simulink model "ProgrammingCalculator"  (R2021a)
settings: Solver=FixedStepDiscrete  StartTime=0.0  StopTime=10.0  RelTol=1e-3  EnableMultiTasking=on
libraries: simulink x6
settings Model: Creator=top one  LastModifiedBy=top one
settings DataIOCC: ReturnWorkspaceOutputs=off
settings OptimizationCC: DefaultParameterBehavior=Inlined  InlineInvariantSignals=on  EnableMemcpy=off  LifeSpan=1  EfficientTunableParamExpr=on
settings DebuggingCC: UnderspecifiedInitializationDetection=Classic  MergeDetectMultiDrivingBlocksExec=none  SFMachineParentedDataDiag=warning  ArithmeticOperatorsInVariantConditions=warning
settings ModelReferenceCC: PropagateSignalLabelsOutOfModel=off
settings SFSimCC: MATLABDynamicMemAlloc=off  CustomCodeUndefinedFunction=UseInterfaceOnly
settings RTWCC: SystemTargetFile=ert.tlc  GenCodeOnly=on  TemplateMakefile=ert_default_tmf  GenerateReport=on  IncludeHyperlinkInReport=on  LaunchReport=on  GenerateTraceInfo=on  GenerateTraceReport=on  GenerateTraceReportSl=on  GenerateTraceReportSf=on  GenerateTraceReportEml=on
settings CodeAppCC: ForceParamTrailComments=on  IgnoreCustomStorageClasses=off  OperatorAnnotations=on  SimulinkDataObjDesc=on  SFDataObjDesc=on  MATLABFcnDesc=on  InsertBlockDesc=on  StateflowObjectComments=on  MATLABSourceComments=on
settings ERTTargetCC: MultiwordLength=2048  GenerateSampleERTMain=on  InlinedParameterPlacement=NonHierarchical  ERTCustomFileTemplate=example_file_process.tlc

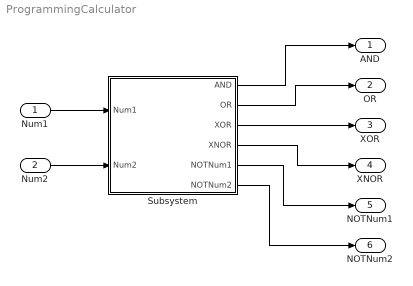
== system ProgrammingCalculator ==
  Num1 : Inport
  Num2 : Inport  Port=2
  Subsystem : Subsystem
  AND : Outport
  OR : Outport  Port=2
  XOR : Outport  Port=3
  XNOR : Outport  Port=4
  NOTNum1 : Outport  Port=5
  NOTNum2 : Outport  Port=6
  wires:
  Subsystem/1(AND) -> AND/1
  Subsystem/2(OR) -> OR/1
  Subsystem/3(XOR) -> XOR/1
  Subsystem/4(XNOR) -> XNOR/1
  Subsystem/5(NOTNum1) -> NOTNum1/1
  Subsystem/6(NOTNum2) -> NOTNum2/1
  Num2/1 -> Subsystem/2(Num2)
  Num1/1 -> Subsystem/1(Num1)

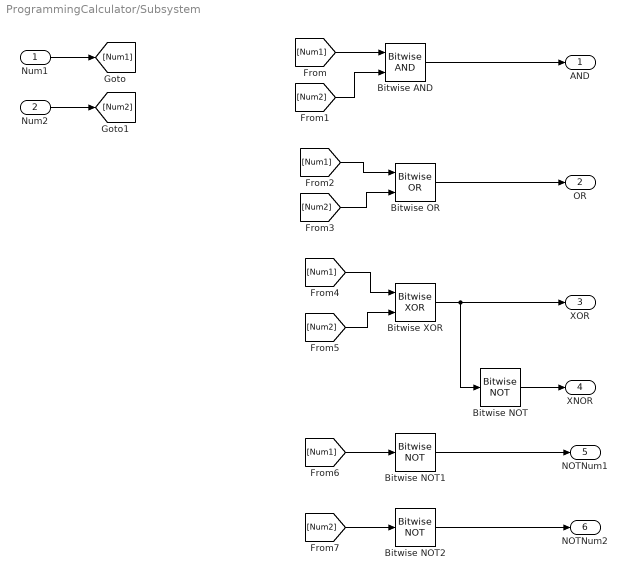
== system ProgrammingCalculator/Subsystem ==
  Num1 : Inport  OutDataTypeStr=uint8
  Num2 : Inport  Port=2  OutDataTypeStr=uint8
  Bitwise AND : simulink/Logic and Bit Operations/Bitwise Operator  logicop=AND  UseBitMask=off  NumInputPorts=2  BitMask=bin2dec('11011001')  BitMaskRealWorld=Stored Integer
  Bitwise NOT : simulink/Logic and Bit Operations/Bitwise Operator  logicop=NOT  UseBitMask=off  BitMask=bin2dec('11011001')  BitMaskRealWorld=Stored Integer
  Bitwise NOT1 : simulink/Logic and Bit Operations/Bitwise Operator  logicop=NOT  UseBitMask=off  BitMask=bin2dec('11011001')  BitMaskRealWorld=Stored Integer
  Bitwise NOT2 : simulink/Logic and Bit Operations/Bitwise Operator  logicop=NOT  UseBitMask=off  BitMask=bin2dec('11011001')  BitMaskRealWorld=Stored Integer
  Bitwise OR : simulink/Logic and Bit Operations/Bitwise Operator  logicop=OR  UseBitMask=off  NumInputPorts=2  BitMask=bin2dec('11011001')  BitMaskRealWorld=Stored Integer
  Bitwise XOR : simulink/Logic and Bit Operations/Bitwise Operator  logicop=XOR  UseBitMask=off  NumInputPorts=2  BitMask=bin2dec('11011001')  BitMaskRealWorld=Stored Integer
  AND : Outport
  OR : Outport  Port=2
  XOR : Outport  Port=3
  XNOR : Outport  Port=4
  NOTNum1 : Outport  Port=5
  NOTNum2 : Outport  Port=6
  wires:
  Num1/1 -> [Num1]
  Bitwise XOR/1 -> XOR/1, Bitwise NOT/1
  [Num2] -> Bitwise XOR/2
  [Num1] -> Bitwise AND/1
  [Num1] -> Bitwise XOR/1
  [Num1] -> Bitwise OR/1
  [Num2] -> Bitwise NOT2/1
  [Num1] -> Bitwise NOT1/1
  Num2/1 -> [Num2]
  [Num2] -> Bitwise OR/2
  Bitwise NOT2/1 -> NOTNum2/1
  Bitwise OR/1 -> OR/1
  [Num2] -> Bitwise AND/2
  Bitwise NOT1/1 -> NOTNum1/1
  Bitwise NOT/1 -> XNOR/1
  Bitwise AND/1 -> AND/1
